simulink model "hw3_4"  (R2023a)
settings: Solver=VariableStepAuto  StartTime=0.0  StopTime=10.0  RelTol=1e-3
settings Model: Creator=마이컴  LastModifiedBy=마이컴

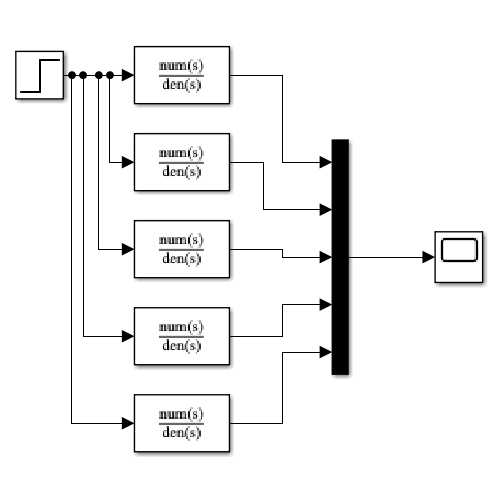
[thumbnail: Simulink's stored preview of the top-level diagram]
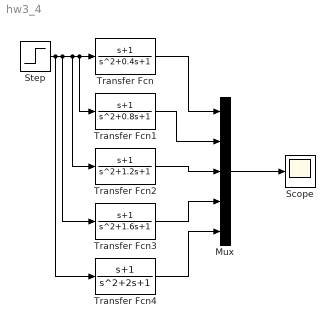
== system hw3_4 ==
  Mux : Mux  Inputs=5
  Scope : Scope
  Step : Step  SampleTime=0
  Transfer Fcn : TransferFcn  Numerator=[1 1]  Denominator=[1 0.4 1]
  Transfer Fcn1 : TransferFcn  Numerator=[1 1]  Denominator=[1 0.8 1]
  Transfer Fcn2 : TransferFcn  Numerator=[1 1]  Denominator=[1 1.2 1]
  Transfer Fcn3 : TransferFcn  Numerator=[1 1]  Denominator=[1 1.6 1]
  Transfer Fcn4 : TransferFcn  Numerator=[1 1]
  wires:
  Step/1 -> Transfer Fcn4/1, Transfer Fcn3/1, Transfer Fcn2/1, Transfer Fcn1/1, Transfer Fcn/1
  Transfer Fcn/1 -> Mux/1
  Transfer Fcn1/1 -> Mux/2
  Transfer Fcn2/1 -> Mux/3
  Transfer Fcn3/1 -> Mux/4
  Transfer Fcn4/1 -> Mux/5
  Mux/1 -> Scope/1
